simulink model "gm_smartCart3"  (R2016a)
settings: Solver=FixedStepDiscrete  StartTime=0.0  StopTime=600000  FixedStep=1  RelTol=1e-3
libraries: simulink x56, hdlsllib x28
(part 1 of 2)
settings Model: Creator=Admin  LastModifiedBy=Admin
settings OptimizationCC: BlockReduction=off  ConditionallyExecuteInputs=off  DefaultParameterBehavior=Inlined
settings DebuggingCC: AlgebraicLoopMsg=error  InheritedTsInSrcMsg=none
settings HardwareCC: ProdBitPerPointer=32  ProdLargestAtomicFloat=None  ProdIntDivRoundTo=Undefined  ProdEndianess=Unspecified  ProdWordSize=32  ProdHWDeviceType=ASIC/FPGA->ASIC/FPGA  ProdEqTarget=off

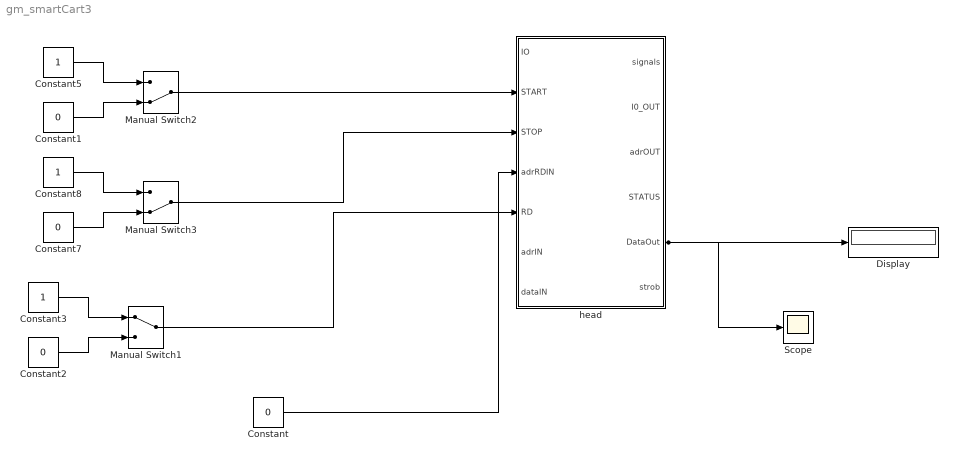
== system gm_smartCart3 ==
  Constant : Constant  Value=0  OutDataTypeStr=uint8
  Constant1 : Constant  Value=0  OutDataTypeStr=boolean
  Constant2 : Constant  Value=0  OutDataTypeStr=boolean
  Constant3 : Constant  OutDataTypeStr=boolean
  Constant5 : Constant  OutDataTypeStr=boolean
  Constant7 : Constant  Value=0  OutDataTypeStr=boolean
  Constant8 : Constant  OutDataTypeStr=boolean
  Display : Display
  Manual Switch1 : ManualSwitch
  Manual Switch2 : ManualSwitch  CurrentSetting=0
  Manual Switch3 : ManualSwitch  CurrentSetting=0
  Scope : Scope
  head : Subsystem  TreatAsAtomicUnit=on
  wires:
  Manual Switch1/1 -> head/5(RD)
  head/5(DataOut) -> Display/1, Scope/1
  Constant2/1 -> Manual Switch1/2
  Constant3/1 -> Manual Switch1/1
  Constant/1 -> head/4(adrRDIN)
  Manual Switch3/1 -> head/3(STOP)
  Constant7/1 -> Manual Switch3/2
  Constant8/1 -> Manual Switch3/1
  Manual Switch2/1 -> head/2(START)
  Constant1/1 -> Manual Switch2/2
  Constant5/1 -> Manual Switch2/1

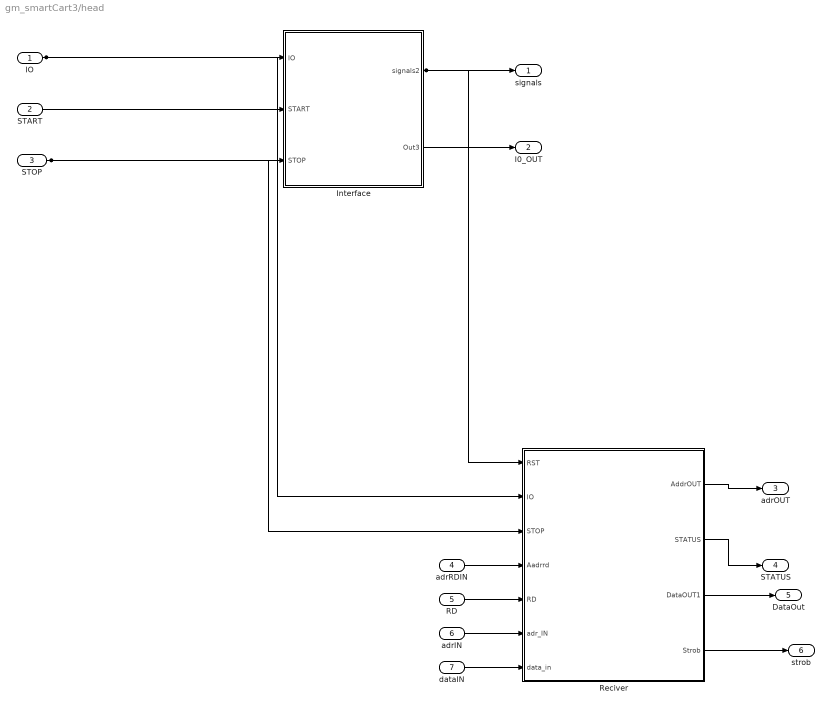
== system gm_smartCart3/head ==
  IO : Inport  OutDataTypeStr=boolean
  START : Inport  Port=2  OutDataTypeStr=boolean  SampleTime=1
  STOP : Inport  Port=3  OutDataTypeStr=boolean  SampleTime=1
  adrRDIN : Inport  Port=4  OutDataTypeStr=uint8
  RD : Inport  Port=5  OutDataTypeStr=boolean  SampleTime=1
  adrIN : Inport  Port=6  OutDataTypeStr=uint8
  dataIN : Inport  Port=7  OutDataTypeStr=uint32
  Interface : Subsystem
  Reciver : Subsystem
  signals : Outport  OutDataTypeStr=fixdt(1,4,0)
  I0_OUT : Outport  Port=2  OutDataTypeStr=boolean
  adrOUT : Outport  Port=3  OutDataTypeStr=uint8
  STATUS : Outport  Port=4  OutDataTypeStr=uint32
  DataOut : Outport  Port=5  OutDataTypeStr=uint8
  strob : Outport  Port=6  OutDataTypeStr=boolean
  wires:
  IO/1 -> Reciver/2(IO), Interface/1(IO)
  START/1 -> Interface/2(START)
  STOP/1 -> Reciver/3(STOP), Interface/3(STOP)
  adrRDIN/1 -> Reciver/4(Aadrrd)
  RD/1 -> Reciver/5(RD)
  adrIN/1 -> Reciver/6(adr_IN)
  dataIN/1 -> Reciver/7(data_in)
  Interface/1(signals2) -> Reciver/1(RST), signals/1
  Interface/2(Out3) -> I0_OUT/1
  Reciver/1(AddrOUT) -> adrOUT/1
  Reciver/2(STATUS) -> STATUS/1
  Reciver/3(DataOUT1) -> DataOut/1
  Reciver/4(Strob) -> strob/1

== system gm_smartCart3/head/Interface ==
  IO : Inport  OutDataTypeStr=boolean
  START : Inport  Port=2  OutDataTypeStr=boolean  SampleTime=1
  STOP : Inport  Port=3  OutDataTypeStr=boolean  SampleTime=1
  ColdStart : Subsystem
  ColdStop2 : Subsystem
  Head2 : Subsystem
  MUX2 : Subsystem
  Swith_signal2 : Subsystem
  signals2 : Outport  OutDataTypeStr=fixdt(1,4,0)  InitialOutput=0
  Out3 : Outport  Port=2  OutDataTypeStr=boolean  InitialOutput=0
  wires:
  IO/1 -> Out3/1, ColdStart/1(Reqest)
  START/1 -> Head2/3(START)
  STOP/1 -> Head2/4(STOP)
  ColdStart/1(DataOUT) -> MUX2/5(DAT_ST1)
  ColdStart/2(Signal) -> MUX2/2(DATA_0)
  ColdStart/3(ADR_OUT) -> MUX2/4(ADR_ST)
  ColdStop2/1(DataOUT) -> MUX2/7(DAT_STOP)
  ColdStop2/2(Signal) -> MUX2/3(DATA_1)
  ColdStop2/3(ADR_OUT) -> MUX2/6(ADR_STOP)
  Head2/1(AdrOut) -> Swith_signal2/1(Adr), ColdStart/2(Addr), ColdStop2/1(Addr)
  Head2/2(DataOut) -> Swith_signal2/2(Data), ColdStart/3(Data), ColdStop2/2(Data)
  MUX2/1(Signals) -> signals2/1
  MUX2/2(ADR_OUT) -> Head2/1(ADR_IN)
  MUX2/3(DATA_OUT1) -> Head2/2(DataIN)
  Swith_signal2/1(OutAddr) -> MUX2/1(ADR)

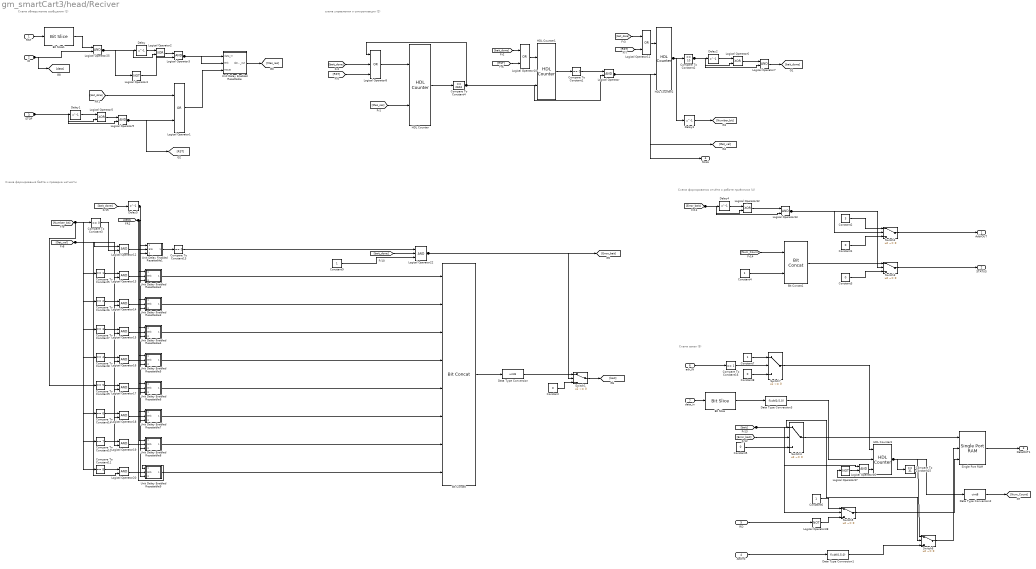
== system gm_smartCart3/head/Reciver ==
  note: Схема обнаружение сообщения (1)
  note: cхема управления и синхронизации (2)
  note: Схема формирования отчёта о работе приёмника (4)
  note: Схема связи (5)
  note: Cхема формирования байта и проверка четности
  RST : Inport  OutDataTypeStr=fixdt(1,4,0)  SampleTime=1
  IO : Inport  Port=2  OutDataTypeStr=boolean
  STOP : Inport  Port=3  OutDataTypeStr=boolean  SampleTime=1
  Aadrrd : Inport  Port=4  OutDataTypeStr=uint8
  RD : Inport  Port=5  OutDataTypeStr=boolean  SampleTime=1
  adr_IN : Inport  Port=6  OutDataTypeStr=uint8
  data_in : Inport  Port=7  OutDataTypeStr=uint32
  Bit Concat : hdlsllib/HDL Operations/Bit Concat  numInputs=8
  Bit Concat1 : hdlsllib/HDL Operations/Bit Concat  numInputs=2
  Bit Slice : hdlsllib/HDL Operations/Bit Slice  lidx=5  ridx=0
  Bit Slice1 : hdlsllib/HDL Operations/Bit Slice  lidx=3  ridx=3
  Compare To Constant1 : simulink/Logic and Bit Operations/Compare To Constant  relop===  const=0  OutDataTypeStr=boolean
  Compare To Constant10 : simulink/Logic and Bit Operations/Compare To Constant  relop===  const=7  OutDataTypeStr=boolean
  Compare To Constant11 : simulink/Logic and Bit Operations/Compare To Constant  relop===  const=8  OutDataTypeStr=boolean
  Compare To Constant13 : simulink/Logic and Bit Operations/Compare To Constant  relop===  const=0  OutDataTypeStr=boolean
  Compare To Constant14 : simulink/Logic and Bit Operations/Compare To Constant  relop===  const=6  OutDataTypeStr=boolean
  Compare To Constant15 : simulink/Logic and Bit Operations/Compare To Constant  relop===  const=31  OutDataTypeStr=boolean
  Compare To Constant16 : simulink/Logic and Bit Operations/Compare To Constant  relop===  const=1  OutDataTypeStr=boolean
  Compare To Constant2 : simulink/Logic and Bit Operations/Compare To Constant  relop===  const=10  OutDataTypeStr=boolean
  Compare To Constant3 : simulink/Logic and Bit Operations/Compare To Constant  relop===  const=0  OutDataTypeStr=boolean
  Compare To Constant4 : simulink/Logic and Bit Operations/Compare To Constant  relop===  const=2604  OutDataTypeStr=boolean
  Compare To Constant5 : simulink/Logic and Bit Operations/Compare To Constant  relop===  const=1  OutDataTypeStr=boolean
  Compare To Constant6 : simulink/Logic and Bit Operations/Compare To Constant  relop===  const=2  OutDataTypeStr=boolean
  Compare To Constant7 : simulink/Logic and Bit Operations/Compare To Constant  relop===  const=3  OutDataTypeStr=boolean
  Compare To Constant8 : simulink/Logic and Bit Operations/Compare To Constant  relop===  const=4  OutDataTypeStr=boolean
  Compare To Constant9 : simulink/Logic and Bit Operations/Compare To Constant  relop===  const=5  OutDataTypeStr=boolean
  Constant : Constant  Value=0  OutDataTypeStr=uint8
  Constant1 : Constant  Value=0  OutDataTypeStr=uint8
  Constant2 : Constant  Value=3  OutDataTypeStr=uint8
  Constant3 : Constant  Value=0  OutDataTypeStr=uint32
  Constant4 : Constant  OutDataTypeStr=boolean
  Constant5 : Constant  Value=0  OutDataTypeStr=uint8  SampleTime=-1
  Constant6 : Constant  OutDataTypeStr=boolean  SampleTime=-1
  Constant7 : Constant  OutDataTypeStr=boolean
  Constant8 : Constant  Value=0  OutDataTypeStr=boolean
  Constant9 : Constant  OutDataTypeStr=boolean
  Data Type Conversion : DataTypeConversion  OutDataTypeStr=uint8
  Data Type Conversion1 : DataTypeConversion  OutDataTypeStr=fixdt(0,5,0)
  Data Type Conversion2 : DataTypeConversion  OutDataTypeStr=uint8
  Data Type Conversion3 : DataTypeConversion  OutDataTypeStr=fixdt(0,5,0)
  Delay{,1..5} (6 alike) : Delay  DelayLength=1  InitialCondition=0
  HDL Counter : hdlsllib/HDL Operations/HDL Counter  CountType=Free running  CountInit=0  CountStep=1  CountMax=1  CountFromType=Initial value  CountFrom=0  CountResetPort=on  CountLoadPort=off  CountEnbPort=on  CountDirPort=off  CountDataType=Unsigned  CountWordLen=13  CountFracLen=0  CountSampTime=1
  HDL Counter1 : hdlsllib/HDL Operations/HDL Counter  CountType=Free running  CountInit=0  CountStep=1  CountMax=1  CountFromType=Initial value  CountFrom=0  CountResetPort=on  CountLoadPort=off  CountEnbPort=on  CountDirPort=off  CountDataType=Unsigned  CountWordLen=1  CountFracLen=0  CountSampTime=1
  HDL Counter2 : hdlsllib/HDL Operations/HDL Counter  CountType=Count limited  CountInit=0  CountStep=1  CountMax=10  CountFromType=Initial value  CountFrom=0  CountResetPort=on  CountLoadPort=off  CountEnbPort=on  CountDirPort=off  CountDataType=Unsigned  CountWordLen=4  CountFracLen=0  CountSampTime=1
  HDL Counter3 : hdlsllib/HDL Operations/HDL Counter  CountType=Free running  CountInit=0  CountStep=1  CountMax=1  CountFromType=Initial value  CountFrom=0  CountResetPort=off  CountLoadPort=on  CountEnbPort=on  CountDirPort=off  CountDataType=Unsigned  CountWordLen=5  CountFracLen=0  CountSampTime=1
  Logical Operator{,3,7,9,12..20,25,33,36} (16 alike) : Logic  AllPortsSameDT=off  OutDataTypeStr=boolean
  Logical Operator1 : Logic  Operator=OR  AllPortsSameDT=off  OutDataTypeStr=boolean
  Logical Operator10 : Logic  Operator=OR  AllPortsSameDT=off  OutDataTypeStr=boolean
  Logical Operator11 : Logic  Operator=OR  AllPortsSameDT=off  OutDataTypeStr=boolean
  Logical Operator{2,5..6,32} (4 alike) : Logic  Operator=XOR  AllPortsSameDT=off  OutDataTypeStr=boolean
  Logical Operator22 : Logic  Inputs=3  AllPortsSameDT=off  OutDataTypeStr=boolean
  Logical Operator37 : Logic  Operator=NOT  AllPortsSameDT=off  OutDataTypeStr=boolean
  Logical Operator38 : Logic  Operator=NOT  AllPortsSameDT=off  OutDataTypeStr=boolean
  Logical Operator4 : Logic  Operator=NOT  AllPortsSameDT=off  OutDataTypeStr=boolean
  Logical Operator8 : Logic  Operator=OR  Inputs=3  AllPortsSameDT=off  OutDataTypeStr=boolean
  Single Port RAM : hdlsllib/HDL Operations/Single Port RAM  ram_size=5  dout_type=Old data
  Switch{1..7} (7 alike) : Switch  Criteria=u2 ~= 0
  Unit Delay Enabled Resettable : Subsystem
  Unit Delay Enabled Resettable1 : Subsystem
  Unit Delay Enabled Resettable2 : Subsystem
  Unit Delay Enabled Resettable3 : Subsystem
  Unit Delay Enabled Resettable4 : Subsystem
  Unit Delay Enabled Resettable5 : Subsystem
  Unit Delay Enabled Resettable6 : Subsystem
  Unit Delay Enabled Resettable7 : Subsystem
  Unit Delay Enabled Resettable8 : Subsystem
  Unit Delay Enabled Resettable9 : Subsystem
  AddrOUT : Outport  OutDataTypeStr=uint8
  STATUS : Outport  Port=2  OutDataTypeStr=uint32
  DataOUT1 : Outport  Port=3  OutDataTypeStr=uint8
  Strob : Outport  Port=4  OutDataTypeStr=boolean
  wires:
  RST/1 -> Bit Slice1/1
  IO/1 -> Logical Operator25/2, [data]
  STOP/1 -> Logical Operator9/2, Logical Operator5/2, Delay1/1
  Aadrrd/1 -> Data Type Conversion1/1
  RD/1 -> Logical Operator38/1
  adr_IN/1 -> Compare To Constant16/1
  data_in/1 -> Bit Slice/1
  Bit Concat/1 -> Data Type Conversion/1
  Bit Concat1/1 -> Switch3/1
  Bit Slice/1 -> Data Type Conversion3/1
  Bit Slice1/1 -> Logical Operator25/1
  Compare To Constant1/1 -> Logical Operator/1
  Compare To Constant10/1 -> Logical Operator19/1
  Compare To Constant11/1 -> Logical Operator20/1
  Compare To Constant13/1 -> Logical Operator22/1
  Compare To Constant14/1 -> Logical Operator18/1
  Compare To Constant15/1 -> Logical Operator37/1
  Compare To Constant16/1 -> Switch7/2
  Compare To Constant2/1 -> Logical Operator7/2, Logical Operator6/2, Delay2/1
  Compare To Constant3/1 -> Logical Operator12/2
  Compare To Constant4/1 -> Logical Operator8/1, Logical Operator/2, HDL Counter1/2
  Compare To Constant5/1 -> Logical Operator13/1
  Compare To Constant6/1 -> Logical Operator14/1
  Compare To Constant7/1 -> Logical Operator15/1
  Compare To Constant8/1 -> Logical Operator16/1
  Compare To Constant9/1 -> Logical Operator17/1
  Constant/1 -> Switch1/3
  Constant1/1 -> Switch2/3
  Constant2/1 -> Switch2/1
  Constant3/1 -> Switch3/3
  Constant4/1 -> Bit Concat1/2
  Constant5/1 -> Switch4/3
  Constant6/1 -> Switch5/1
  Constant7/1 -> Switch7/1
  Constant8/1 -> Switch7/3
  Constant9/1 -> Logical Operator22/3
  Data Type Conversion/1 -> Switch1/1
  Data Type Conversion1/1 -> Switch6/3
  Data Type Conversion2/1 -> [Num_Count]
  Data Type Conversion3/1 -> HDL Counter3/2
  Delay/1 -> Logical Operator2/1
  Delay1/1 -> Logical Operator5/1
  Delay2/1 -> Logical Operator6/1
  Delay3/1 -> [Number_bit]
  Delay4/1 -> Logical Operator32/1
  Delay5/1 -> Unit Delay Enabled Resettable9/3(Reset), Unit Delay Enabled Resettable8/3(Reset), Unit Delay Enabled Resettable7/3(Reset), Unit Delay Enabled Resettable6/3(Reset), Unit Delay Enabled Resettable5/3(Reset), Unit Delay Enabled Resettable4/3(Reset), Unit Delay Enabled Resettable3/3(Reset), Unit Delay Enabled Resettable2/3(Reset), Unit Delay Enabled Resettable1/3(Reset)
  [bait_done] -> Logical Operator1/1
  [data] -> Unit Delay Enabled Resettable9/1(data_in), Unit Delay Enabled Resettable8/1(data_in), Unit Delay Enabled Resettable7/1(data_in), Unit Delay Enabled Resettable6/1(data_in), Unit Delay Enabled Resettable5/1(data_in), Unit Delay Enabled Resettable4/1(data_in), Unit Delay Enabled Resettable3/1(data_in), Unit Delay Enabled Resettable2/1(data_in), Unit Delay Enabled Resettable1/1(data_in)
  [Mes_res] -> HDL Counter/2
  [bait_done] -> Logical Operator22/2
  [Error_bait] -> Logical Operator33/2, Logical Operator32/2, Delay4/1
  [Error_bait] -> Switch4/2
  [bait] -> Switch6/2, Switch5/2, Switch4/1, Logical Operator36/1
  [Num_Count] -> Bit Concat1/1
  [bait_done] -> Delay5/1
  [bait_done] -> Logical Operator10/1
  [bait_done] -> Logical Operator11/1
  [bait_done] -> Logical Operator8/2
  [RST] -> Logical Operator8/3
  [RST] -> Logical Operator10/2
  [RST] -> Logical Operator11/2
  [Get_val] -> Logical Operator20/2, Logical Operator19/2, Logical Operator18/2, Logical Operator17/2, Logical Operator16/2, Logical Operator15/2, Logical Operator14/2, Logical Operator13/2, Logical Operator12/1
  [Number_bit] -> Compare To Constant9/1, Compare To Constant8/1, Compare To Constant7/1, Compare To Constant6/1, Compare To Constant5/1, Compare To Constant3/1, Compare To Constant14/1, Compare To Constant11/1, Compare To Constant10/1
  HDL Counter/1 -> Compare To Constant4/1
  HDL Counter1/1 -> Compare To Constant1/1
  HDL Counter2/1 -> Compare To Constant2/1, Delay3/1
  HDL Counter3/1 -> Switch6/1, Data Type Conversion2/1, Compare To Constant15/1
  Logical Operator/1 -> HDL Counter2/2, [Get_val], Strob/1
  Logical Operator1/1 -> Unit Delay Enabled Resettable/3(Reset)
  Logical Operator10/1 -> HDL Counter1/1
  Logical Operator11/1 -> HDL Counter2/1
  Logical Operator12/1 -> Unit Delay Enabled Resettable1/2(Enb)
  Logical Operator13/1 -> Unit Delay Enabled Resettable2/2(Enb)
  Logical Operator14/1 -> Unit Delay Enabled Resettable3/2(Enb)
  Logical Operator15/1 -> Unit Delay Enabled Resettable4/2(Enb)
  Logical Operator16/1 -> Unit Delay Enabled Resettable5/2(Enb)
  Logical Operator17/1 -> Unit Delay Enabled Resettable6/2(Enb)
  Logical Operator18/1 -> Unit Delay Enabled Resettable7/2(Enb)
  Logical Operator19/1 -> Unit Delay Enabled Resettable8/2(Enb)
  Logical Operator2/1 -> Logical Operator3/1
  Logical Operator20/1 -> Unit Delay Enabled Resettable9/2(Enb)
  Logical Operator22/1 -> Switch1/2, [Error_bait]
  Logical Operator25/1 -> Logical Operator4/1, Logical Operator2/2, Delay/1
  Logical Operator3/1 -> Unit Delay Enabled Resettable/2(Enb), Unit Delay Enabled Resettable/1(data_in)
  Logical Operator32/1 -> Logical Operator33/1
  Logical Operator33/1 -> Switch3/2, Switch2/2
  Logical Operator36/1 -> HDL Counter3/3
  Logical Operator37/1 -> Logical Operator36/2
  Logical Operator38/1 -> Switch5/3
  Logical Operator4/1 -> Logical Operator3/2
  Logical Operator5/1 -> Logical Operator9/1
  Logical Operator6/1 -> Logical Operator7/1
  Logical Operator7/1 -> [bait_done]
  Logical Operator8/1 -> HDL Counter/1
  Logical Operator9/1 -> Logical Operator1/2, [RST]
  Single Port RAM/1 -> DataOUT1/1
  Switch1/1 -> [bait]
  Switch2/1 -> AddrOUT/1
  Switch3/1 -> STATUS/1
  Switch4/1 -> Single Port RAM/1
  Switch5/1 -> Single Port RAM/3
  Switch6/1 -> Single Port RAM/2
  Switch7/1 -> HDL Counter3/1
  Unit Delay Enabled Resettable/1(data_out) -> [Mes_res]
  Unit Delay Enabled Resettable1/1(data_out) -> Compare To Constant13/1
  Unit Delay Enabled Resettable2/1(data_out) -> Bit Concat/1
  Unit Delay Enabled Resettable3/1(data_out) -> Bit Concat/2
  Unit Delay Enabled Resettable4/1(data_out) -> Bit Concat/3
  Unit Delay Enabled Resettable5/1(data_out) -> Bit Concat/4
  Unit Delay Enabled Resettable6/1(data_out) -> Bit Concat/5
  Unit Delay Enabled Resettable7/1(data_out) -> Bit Concat/6
  Unit Delay Enabled Resettable8/1(data_out) -> Bit Concat/7
  Unit Delay Enabled Resettable9/1(data_out) -> Bit Concat/8

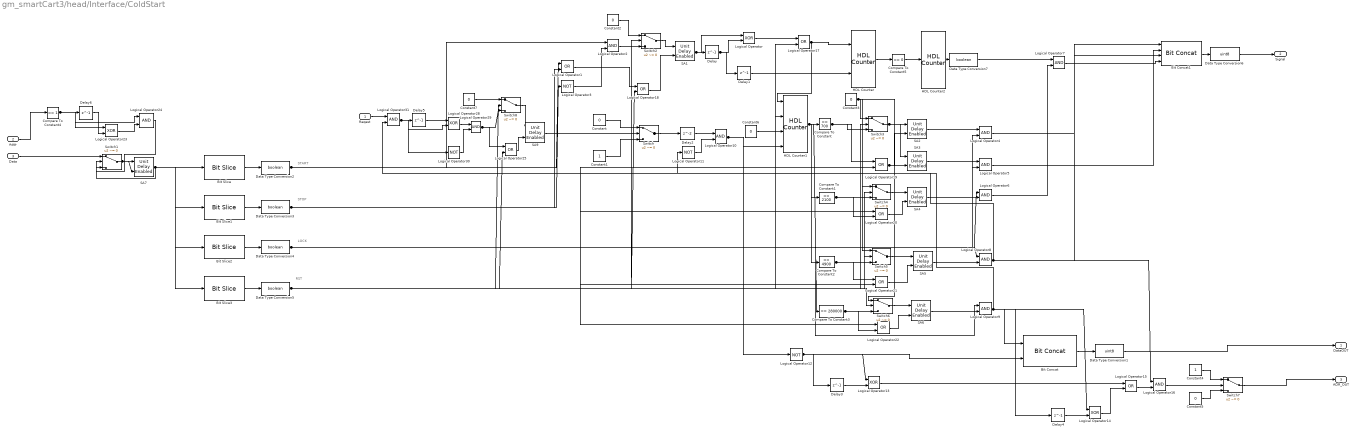
== system gm_smartCart3/head/Interface/ColdStart ==
  note: LOCK
  note: STOP
  note: START
  note: RST
  Reqest : Inport  OutDataTypeStr=boolean
  Addr : Inport  Port=2  OutDataTypeStr=uint8  SampleTime=1
  Data : Inport  Port=3  OutDataTypeStr=uint8  SampleTime=1
  Bit Concat : hdlsllib/HDL Operations/Bit Concat  numInputs=2
  Bit Concat1 : hdlsllib/HDL Operations/Bit Concat  numInputs=4
  Bit Slice : hdlsllib/HDL Operations/Bit Slice  lidx=3  ridx=3
  Bit Slice1 : hdlsllib/HDL Operations/Bit Slice  lidx=2  ridx=2
  Bit Slice2 : hdlsllib/HDL Operations/Bit Slice  lidx=1  ridx=1
  Bit Slice3 : hdlsllib/HDL Operations/Bit Slice  lidx=0  ridx=0
  Compare To Constant : simulink/Logic and Bit Operations/Compare To Constant  relop===  const=700  OutDataTypeStr=boolean
  Compare To Constant1 : simulink/Logic and Bit Operations/Compare To Constant  relop===  const=2100  OutDataTypeStr=boolean
  Compare To Constant2 : simulink/Logic and Bit Operations/Compare To Constant  relop===  const=4900  OutDataTypeStr=boolean
  Compare To Constant3 : simulink/Logic and Bit Operations/Compare To Constant  relop===  const=280000  OutDataTypeStr=boolean
  Compare To Constant4 : simulink/Logic and Bit Operations/Compare To Constant  relop===  const=1  OutDataTypeStr=boolean
  Compare To Constant5 : simulink/Logic and Bit Operations/Compare To Constant  relop===  const=0  OutDataTypeStr=boolean
  Constant{,2..3,7} (4 alike) : Constant  Value=0  OutDataTypeStr=boolean
  Constant1 : Constant  OutDataTypeStr=boolean
  Constant4 : Constant  OutDataTypeStr=uint8
  Constant5 : Constant  Value=0  OutDataTypeStr=uint8
  Constant6 : Constant  Value=0  OutDataTypeStr=fixdt(0,32,0)
  Data Type Conversion1 : DataTypeConversion  OutDataTypeStr=uint8
  Data Type Conversion{2..5,7} (5 alike) : DataTypeConversion  OutDataTypeStr=boolean
  Data Type Conversion6 : DataTypeConversion  OutDataTypeStr=uint8
  Delay{,1,3..6} (6 alike) : Delay  DelayLength=1  InitialCondition=0
  Delay2 : Delay  InitialCondition=0
  HDL Counter : hdlsllib/HDL Operations/HDL Counter  CountType=Count limited  CountInit=0  CountStep=1  CountMax=6  CountFromType=Initial value  CountFrom=0  CountResetPort=on  CountLoadPort=off  CountEnbPort=on  CountDirPort=off  CountDataType=Unsigned  CountWordLen=3  CountFracLen=0  CountSampTime=277e-9
  HDL Counter1 : hdlsllib/HDL Operations/HDL Counter  CountType=Count limited  CountInit=0  CountStep=1  CountMax=40000  CountFromType=Initial value  CountFrom=0  CountResetPort=on  CountLoadPort=on  CountEnbPort=on  CountDirPort=off  CountDataType=Unsigned  CountWordLen=32  CountFracLen=0  CountSampTime=277e-9
  HDL Counter2 : hdlsllib/HDL Operations/HDL Counter  CountType=Free running  CountInit=0  CountStep=1  CountMax=5  CountFromType=Initial value  CountFrom=0  CountResetPort=off  CountLoadPort=off  CountEnbPort=on  CountDirPort=off  CountDataType=Unsigned  CountWordLen=1  CountFracLen=0  CountSampTime=277e-9
  Logical Operator{,13..14,23,28} (5 alike) : Logic  Operator=XOR  AllPortsSameDT=off  OutDataTypeStr=boolean
  Logical Operator{1,15,17..22,25} (9 alike) : Logic  Operator=OR  AllPortsSameDT=off  OutDataTypeStr=boolean
  Logical Operator{2,4..10,16,24,29,31} (12 alike) : Logic  AllPortsSameDT=off  OutDataTypeStr=boolean
  Logical Operator{3,11..12,30} (4 alike) : Logic  Operator=NOT  AllPortsSameDT=off  OutDataTypeStr=boolean
  SA{1..7,9} (8 alike) : simulink/Additional Math & Discrete/Additional Discrete/Unit Delay Enabled  vinit=0  tsamp=-1
  Switch{,1..8} (9 alike) : Switch  Criteria=u2 ~= 0
  DataOUT : Outport  OutDataTypeStr=uint8
  Signal : Outport  Port=2  OutDataTypeStr=uint8
  ADR_OUT : Outport  Port=3  OutDataTypeStr=uint8
  wires:
  Reqest/1 -> Logical Operator31/1
  Addr/1 -> Compare To Constant4/1
  Data/1 -> Switch1/1
  Bit Concat/1 -> Data Type Conversion1/1
  Bit Concat1/1 -> Data Type Conversion6/1
  Bit Slice/1 -> Data Type Conversion2/1
  Bit Slice1/1 -> Data Type Conversion3/1
  Bit Slice2/1 -> Data Type Conversion4/1
  Bit Slice3/1 -> Data Type Conversion5/1
  Compare To Constant/1 -> Switch3/3, Logical Operator19/1
  Compare To Constant1/1 -> Switch4/3, Logical Operator20/2
  Compare To Constant2/1 -> Switch5/3, Logical Operator21/1
  Compare To Constant3/1 -> Switch6/3, Logical Operator22/2
  Compare To Constant4/1 -> Logical Operator24/1, Logical Operator23/1, Delay6/1
  Compare To Constant5/1 -> HDL Counter2/1
  Constant/1 -> Switch/1
  Constant1/1 -> Switch/3
  Constant2/1 -> Switch2/1
  Constant3/1 -> Switch6/1, Switch5/1, Switch4/1, Switch3/1
  Constant4/1 -> Switch7/1
  Constant5/1 -> Switch7/3
  Constant6/1 -> HDL Counter1/3
  Constant7/1 -> Switch8/1
  Data Type Conversion1/1 -> DataOUT/1
  Data Type Conversion2/1 -> Logical Operator2/1, Logical Operator1/1
  Data Type Conversion3/1 -> Logical Operator3/1, Logical Operator1/2
  Data Type Conversion4/1 -> Logical Operator9/1, Logical Operator8/1, Logical Operator6/1, Logical Operator5/2, Logical Operator4/2
  Data Type Conversion5/1 -> Switch8/2, Switch6/2, Switch5/2, Switch4/2, Switch3/2, Switch2/2, Logical Operator25/2, Logical Operator22/1, Logical Operator21/2, Logical Operator20/1, Logical Operator19/2, Logical Operator18/2, Logical Operator17/2, HDL Counter1/2
  Data Type Conversion6/1 -> Signal/1
  Data Type Conversion7/1 -> Logical Operator7/1
  Delay/1 -> Logical Operator/2, Delay1/1
  Delay1/1 -> HDL Counter/2
  Delay2/1 -> Logical Operator10/1
  Delay3/1 -> Logical Operator13/2
  Delay4/1 -> Logical Operator14/2
  Delay5/1 -> Logical Operator28/1
  Delay6/1 -> Logical Operator23/2
  HDL Counter/1 -> Compare To Constant5/1
  HDL Counter1/1 -> Compare To Constant3/1, Compare To Constant2/1, Compare To Constant1/1, Compare To Constant/1
  HDL Counter2/1 -> Data Type Conversion7/1
  Logical Operator/1 -> Logical Operator17/1
  Logical Operator1/1 -> Logical Operator18/1
  Logical Operator10/1 -> Logical Operator12/1, HDL Counter1/4
  Logical Operator11/1 -> Logical Operator10/2
  Logical Operator12/1 -> Logical Operator13/1, Bit Concat/2, Delay3/1
  Logical Operator13/1 -> Logical Operator15/1
  Logical Operator14/1 -> Logical Operator15/2
  Logical Operator15/1 -> Logical Operator16/2
  Logical Operator16/1 -> Switch7/2
  Logical Operator17/1 -> HDL Counter1/1, HDL Counter/1
  Logical Operator18/1 -> SA1/2
  Logical Operator19/1 -> SA3/2, SA2/2
  Logical Operator2/1 -> Switch2/3
  Logical Operator20/1 -> SA4/2
  Logical Operator21/1 -> SA5/2
  Logical Operator22/1 -> SA6/2
  Logical Operator23/1 -> Logical Operator24/2
  Logical Operator24/1 -> Switch1/2
  Logical Operator25/1 -> SA9/2
  Logical Operator28/1 -> Logical Operator29/1
  Logical Operator29/1 -> Switch8/3, Logical Operator25/1
  Logical Operator3/1 -> Logical Operator2/2
  Logical Operator30/1 -> Logical Operator29/2
  Logical Operator31/1 -> Logical Operator30/1, Logical Operator28/2, Delay5/1
  Logical Operator4/1 -> Bit Concat1/3
  Logical Operator5/1 -> Bit Concat1/2
  Logical Operator6/1 -> Logical Operator7/2
  Logical Operator7/1 -> Bit Concat1/4
  Logical Operator8/1 -> Logical Operator31/2, Logical Operator16/1, Bit Concat1/1
  Logical Operator9/1 -> Logical Operator14/1, Logical Operator11/1, Bit Concat/1, Delay4/1
  SA1/1 -> Logical Operator/1, Delay/1
  SA2/1 -> Logical Operator4/1
  SA3/1 -> Logical Operator5/1
  SA4/1 -> Logical Operator6/2
  SA5/1 -> Logical Operator8/2
  SA6/1 -> Logical Operator9/2
  SA7/1 -> Switch1/3, Bit Slice3/1, Bit Slice2/1, Bit Slice1/1, Bit Slice/1
  SA9/1 -> Switch/2
  Switch/1 -> Delay2/1
  Switch1/1 -> SA7/2, SA7/1
  Switch2/1 -> SA1/1
  Switch3/1 -> SA3/1, SA2/1
  Switch4/1 -> SA4/1
  Switch5/1 -> SA5/1
  Switch6/1 -> SA6/1
  Switch7/1 -> ADR_OUT/1
  Switch8/1 -> SA9/1

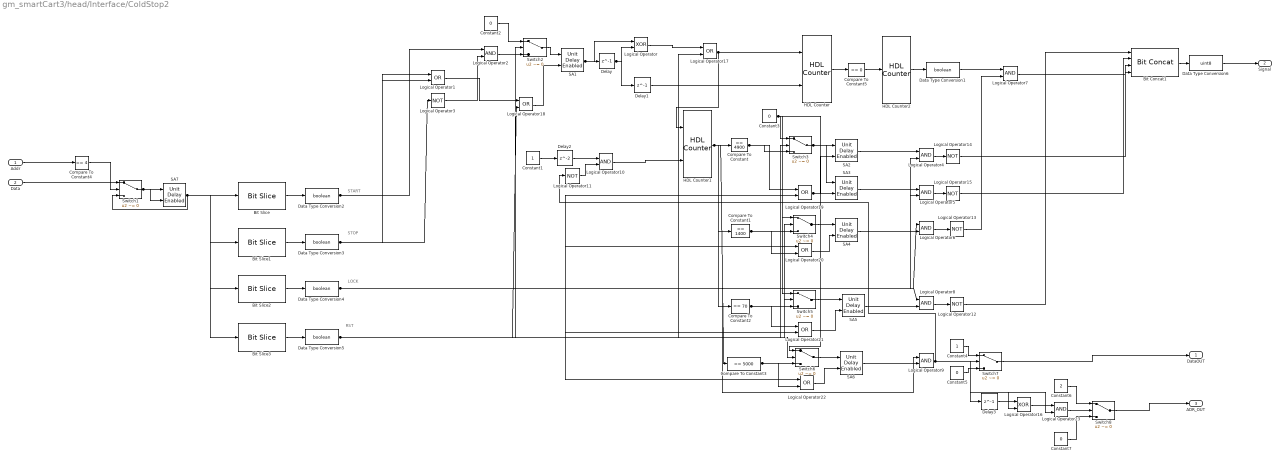
== system gm_smartCart3/head/Interface/ColdStop2 ==
  note: LOCK
  note: STOP
  note: START
  note: RST
  Addr : Inport  OutDataTypeStr=uint8  SampleTime=1
  Data : Inport  Port=2  OutDataTypeStr=uint8  SampleTime=1
  Bit Concat1 : hdlsllib/HDL Operations/Bit Concat  numInputs=4
  Bit Slice : hdlsllib/HDL Operations/Bit Slice  lidx=3  ridx=3
  Bit Slice1 : hdlsllib/HDL Operations/Bit Slice  lidx=2  ridx=2
  Bit Slice2 : hdlsllib/HDL Operations/Bit Slice  lidx=1  ridx=1
  Bit Slice3 : hdlsllib/HDL Operations/Bit Slice  lidx=0  ridx=0
  Compare To Constant : simulink/Logic and Bit Operations/Compare To Constant  relop===  const=4900  OutDataTypeStr=boolean
  Compare To Constant1 : simulink/Logic and Bit Operations/Compare To Constant  relop===  const=1400  OutDataTypeStr=boolean
  Compare To Constant2 : simulink/Logic and Bit Operations/Compare To Constant  relop===  const=70  OutDataTypeStr=boolean
  Compare To Constant3 : simulink/Logic and Bit Operations/Compare To Constant  relop===  const=5000  OutDataTypeStr=boolean
  Compare To Constant4 : simulink/Logic and Bit Operations/Compare To Constant  relop===  const=4  OutDataTypeStr=boolean
  Compare To Constant5 : simulink/Logic and Bit Operations/Compare To Constant  relop===  const=0  OutDataTypeStr=boolean
  Constant1 : Constant  OutDataTypeStr=boolean
  Constant2 : Constant  Value=0  OutDataTypeStr=boolean
  Constant3 : Constant  Value=0  OutDataTypeStr=boolean
  Constant4 : Constant  OutDataTypeStr=uint8
  Constant5 : Constant  Value=0  OutDataTypeStr=uint8
  Constant6 : Constant  Value=2  OutDataTypeStr=uint8
  Constant7 : Constant  Value=0  OutDataTypeStr=uint8
  Data Type Conversion{1..5} (5 alike) : DataTypeConversion  OutDataTypeStr=boolean
  Data Type Conversion6 : DataTypeConversion  OutDataTypeStr=uint8
  Delay : Delay  DelayLength=1  InitialCondition=0
  Delay1 : Delay  DelayLength=1  InitialCondition=0
  Delay2 : Delay  InitialCondition=0
  Delay3 : Delay  DelayLength=1  InitialCondition=0
  HDL Counter : hdlsllib/HDL Operations/HDL Counter  CountType=Count limited  CountInit=0  CountStep=1  CountMax=6  CountFromType=Initial value  CountFrom=0  CountResetPort=on  CountLoadPort=off  CountEnbPort=on  CountDirPort=off  CountDataType=Unsigned  CountWordLen=3  CountFracLen=0  CountSampTime=277e-9
  HDL Counter1 : hdlsllib/HDL Operations/HDL Counter  CountType=Count limited  CountInit=0  CountStep=1  CountMax=40000  CountFromType=Initial value  CountFrom=0  CountResetPort=on  CountLoadPort=off  CountEnbPort=on  CountDirPort=off  CountDataType=Unsigned  CountWordLen=32  CountFracLen=0  CountSampTime=277e-9
  HDL Counter2 : hdlsllib/HDL Operations/HDL Counter  CountType=Free running  CountInit=0  CountStep=1  CountMax=6  CountFromType=Initial value  CountFrom=0  CountResetPort=off  CountLoadPort=off  CountEnbPort=on  CountDirPort=off  CountDataType=Unsigned  CountWordLen=1  CountFracLen=0  CountSampTime=277e-9
  Logical Operator : Logic  Operator=XOR  AllPortsSameDT=off  OutDataTypeStr=boolean
  Logical Operator{1,17..22} (7 alike) : Logic  Operator=OR  AllPortsSameDT=off  OutDataTypeStr=boolean
  Logical Operator{2,4..10,23} (9 alike) : Logic  AllPortsSameDT=off  OutDataTypeStr=boolean
  Logical Operator{3,11..15} (6 alike) : Logic  Operator=NOT  AllPortsSameDT=off  OutDataTypeStr=boolean
  Logical Operator16 : Logic  Operator=XOR  AllPortsSameDT=off  OutDataTypeStr=boolean
  SA{1..7} (7 alike) : simulink/Additional Math & Discrete/Additional Discrete/Unit Delay Enabled  vinit=0  tsamp=-1
  Switch{1..8} (8 alike) : Switch  Criteria=u2 ~= 0
  DataOUT : Outport  OutDataTypeStr=uint8
  Signal : Outport  Port=2  OutDataTypeStr=uint8
  ADR_OUT : Outport  Port=3  OutDataTypeStr=uint8
  wires:
  Addr/1 -> Compare To Constant4/1
  Data/1 -> Switch1/1
  Bit Concat1/1 -> Data Type Conversion6/1
  Bit Slice/1 -> Data Type Conversion2/1
  Bit Slice1/1 -> Data Type Conversion3/1
  Bit Slice2/1 -> Data Type Conversion4/1
  Bit Slice3/1 -> Data Type Conversion5/1
  Compare To Constant/1 -> Switch3/3, Logical Operator19/1
  Compare To Constant1/1 -> Switch4/3, Logical Operator20/2
  Compare To Constant2/1 -> Switch5/3, Logical Operator21/1
  Compare To Constant3/1 -> Switch6/3, Logical Operator22/2
  Compare To Constant4/1 -> Switch1/2
  Compare To Constant5/1 -> HDL Counter2/1
  Constant1/1 -> Delay2/1
  Constant2/1 -> Switch2/1
  Constant3/1 -> Switch6/1, Switch5/1, Switch4/1, Switch3/1
  Constant4/1 -> Switch7/1
  Constant5/1 -> Switch7/3
  Constant6/1 -> Switch8/1
  Constant7/1 -> Switch8/3
  Data Type Conversion1/1 -> Logical Operator7/1
  Data Type Conversion2/1 -> Logical Operator2/1, Logical Operator1/1
  Data Type Conversion3/1 -> Logical Operator3/1, Logical Operator1/2
  Data Type Conversion4/1 -> Logical Operator9/1, Logical Operator8/1, Logical Operator6/1, Logical Operator5/2, Logical Operator4/2
  Data Type Conversion5/1 -> Switch6/2, Switch5/2, Switch4/2, Switch3/2, Switch2/2, Logical Operator22/1, Logical Operator21/2, Logical Operator20/1, Logical Operator19/2, Logical Operator18/2, Logical Operator17/2
  Data Type Conversion6/1 -> Signal/1
  Delay/1 -> Logical Operator/2, Delay1/1
  Delay1/1 -> HDL Counter/2
  Delay2/1 -> Logical Operator10/1
  Delay3/1 -> Logical Operator16/1
  HDL Counter/1 -> Compare To Constant5/1
  HDL Counter1/1 -> Compare To Constant3/1, Compare To Constant2/1, Compare To Constant1/1, Compare To Constant/1
  HDL Counter2/1 -> Data Type Conversion1/1
  Logical Operator/1 -> Logical Operator17/1
  Logical Operator1/1 -> Logical Operator18/1
  Logical Operator10/1 -> HDL Counter1/2
  Logical Operator11/1 -> Logical Operator10/2
  Logical Operator12/1 -> Bit Concat1/1
  Logical Operator13/1 -> Logical Operator7/2
  Logical Operator14/1 -> Bit Concat1/3
  Logical Operator15/1 -> Bit Concat1/2
  Logical Operator16/1 -> Logical Operator23/1
  Logical Operator17/1 -> HDL Counter1/1, HDL Counter/1
  Logical Operator18/1 -> SA1/2
  Logical Operator19/1 -> SA3/2, SA2/2
  Logical Operator2/1 -> Switch2/3
  Logical Operator20/1 -> SA4/2
  Logical Operator21/1 -> SA5/2
  Logical Operator22/1 -> SA6/2
  Logical Operator23/1 -> Switch8/2
  Logical Operator3/1 -> Logical Operator2/2
  Logical Operator4/1 -> Logical Operator14/1
  Logical Operator5/1 -> Logical Operator15/1
  Logical Operator6/1 -> Logical Operator13/1
  Logical Operator7/1 -> Bit Concat1/4
  Logical Operator8/1 -> Logical Operator12/1
  Logical Operator9/1 -> Switch7/2, Logical Operator23/2, Logical Operator16/2, Logical Operator11/1, Delay3/1
  SA1/1 -> Logical Operator/1, Delay/1
  SA2/1 -> Logical Operator4/1
  SA3/1 -> Logical Operator5/1
  SA4/1 -> Logical Operator6/2
  SA5/1 -> Logical Operator8/2
  SA6/1 -> Logical Operator9/2
  SA7/1 -> Switch1/3, Bit Slice3/1, Bit Slice2/1, Bit Slice1/1, Bit Slice/1
  Switch1/1 -> SA7/2, SA7/1
  Switch2/1 -> SA1/1
  Switch3/1 -> SA3/1, SA2/1
  Switch4/1 -> SA4/1
  Switch5/1 -> SA5/1
  Switch6/1 -> SA6/1
  Switch7/1 -> DataOUT/1
  Switch8/1 -> ADR_OUT/1

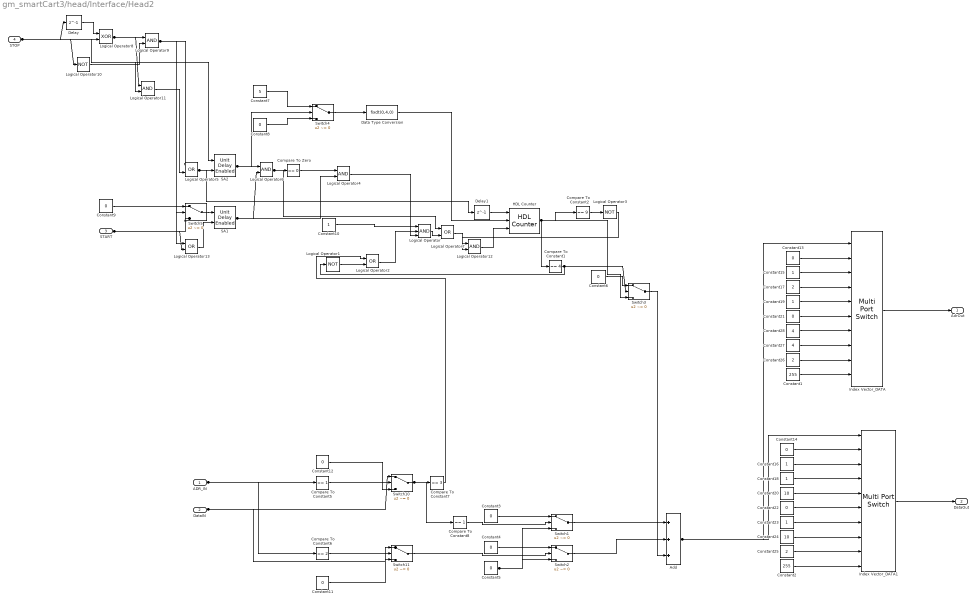
== system gm_smartCart3/head/Interface/Head2 ==
  ADR_IN : Inport  OutDataTypeStr=uint8  SampleTime=1
  DataIN : Inport  Port=2  OutDataTypeStr=uint8  SampleTime=1
  START : Inport  Port=3  OutDataTypeStr=boolean  SampleTime=1
  STOP : Inport  Port=4  OutDataTypeStr=boolean  SampleTime=1
  Add : Sum  Inputs=+++
  Compare To Constant1 : simulink/Logic and Bit Operations/Compare To Constant  relop===  const=4  OutDataTypeStr=boolean
  Compare To Constant2 : simulink/Logic and Bit Operations/Compare To Constant  relop===  const=9  OutDataTypeStr=boolean
  Compare To Constant5 : simulink/Logic and Bit Operations/Compare To Constant  relop===  const=1  OutDataTypeStr=boolean
  Compare To Constant6 : simulink/Logic and Bit Operations/Compare To Constant  relop===  const=2  OutDataTypeStr=boolean
  Compare To Constant7 : simulink/Logic and Bit Operations/Compare To Constant  relop===  const=3  OutDataTypeStr=boolean
  Compare To Constant8 : simulink/Logic and Bit Operations/Compare To Constant  relop===  const=1  OutDataTypeStr=boolean
  Compare To Zero : simulink/Logic and Bit Operations/Compare To Zero  relop===  OutDataTypeStr=boolean
  Constant1 : Constant  Value=255  OutDataTypeStr=uint8
  Constant10 : Constant  OutDataTypeStr=boolean
  Constant{3..6,11..14,21..22} (10 alike) : Constant  Value=0  OutDataTypeStr=uint8
  Constant{15..16,18..19,23} (5 alike) : Constant  OutDataTypeStr=uint8
  Constant17 : Constant  Value=2  OutDataTypeStr=uint8
  Constant2 : Constant  Value=255  OutDataTypeStr=uint8
  Constant20 : Constant  Value=10  OutDataTypeStr=uint8
  Constant24 : Constant  Value=10  OutDataTypeStr=uint8
  Constant25 : Constant  Value=2  OutDataTypeStr=uint8
  Constant26 : Constant  Value=2  OutDataTypeStr=uint8
  Constant27 : Constant  Value=4  OutDataTypeStr=uint8
  Constant28 : Constant  Value=4  OutDataTypeStr=uint8
  Constant7 : Constant  Value=5  OutDataTypeStr=fixdt(0,4,0)
  Constant8 : Constant  Value=0  OutDataTypeStr=fixdt(0,4,0)
  Constant9 : Constant  Value=0  OutDataTypeStr=boolean
  Data Type Conversion : DataTypeConversion  OutDataTypeStr=fixdt(0,4,0)
  Delay : Delay  DelayLength=1  InitialCondition=0
  Delay1 : Delay  DelayLength=1  InitialCondition=0
  HDL Counter : hdlsllib/HDL Operations/HDL Counter  CountType=Free running  CountInit=0  CountStep=1  CountMax=100  CountFromType=Initial value  CountFrom=0  CountResetPort=off  CountLoadPort=on  CountEnbPort=on  CountDirPort=off  CountDataType=Unsigned  CountWordLen=4  CountFracLen=0  CountSampTime=1
  Index Vector_DATA : MultiPortSwitch  DataPortOrder=Zero-based contiguous  Inputs=9  DiagnosticForDefault=None  zeroidx=on  OutDataTypeStr=uint8
  Index Vector_DATA1 : MultiPortSwitch  DataPortOrder=Zero-based contiguous  Inputs=9  DiagnosticForDefault=None  zeroidx=on  OutDataTypeStr=uint8
  Logical Operator : Logic  Inputs=3  AllPortsSameDT=off  OutDataTypeStr=boolean
  Logical Operator1 : Logic  Operator=NOT  AllPortsSameDT=off  OutDataTypeStr=boolean
  Logical Operator10 : Logic  Operator=NOT  AllPortsSameDT=off  OutDataTypeStr=boolean
  Logical Operator{4,6,9,11..12} (5 alike) : Logic  AllPortsSameDT=off  OutDataTypeStr=boolean
  Logical Operator{2,5,7,13} (4 alike) : Logic  Operator=OR  AllPortsSameDT=off  OutDataTypeStr=boolean
  Logical Operator3 : Logic  Operator=NOT  AllPortsSameDT=off  OutDataTypeStr=boolean
  Logical Operator8 : Logic  Operator=XOR  AllPortsSameDT=off  OutDataTypeStr=boolean
  SA1 : simulink/Additional Math & Discrete/Additional Discrete/Unit Delay Enabled  vinit=0  tsamp=-1
  SA2 : simulink/Additional Math & Discrete/Additional Discrete/Unit Delay Enabled  vinit=0  tsamp=-1
  Switch{1..5,10..11} (7 alike) : Switch  Criteria=u2 ~= 0  OutDataTypeStr=uint8
  AdrOut : Outport  OutDataTypeStr=uint8
  DataOut : Outport  Port=2  OutDataTypeStr=uint8
  wires:
  ADR_IN/1 -> Compare To Constant6/1, Compare To Constant5/1
  DataIN/1 -> Switch11/1, Switch10/1
  START/1 -> Switch5/3, Logical Operator13/2
  STOP/1 -> Logical Operator8/2, Logical Operator11/2, Logical Operator10/1, SA2/1, Delay/1
  Add/1 -> Index Vector_DATA1/1, Index Vector_DATA/1
  Compare To Constant1/1 -> Switch3/2, Logical Operator1/1
  Compare To Constant2/1 -> Logical Operator3/1
  Compare To Constant5/1 -> Switch10/2
  Compare To Constant6/1 -> Switch11/2
  Compare To Constant7/1 -> Logical Operator2/1
  Compare To Constant8/1 -> Switch1/2
  Compare To Zero/1 -> Logical Operator4/1
  Constant1/1 -> Index Vector_DATA/10
  Constant10/1 -> Logical Operator/1
  Constant11/1 -> Switch11/3
  Constant12/1 -> Switch10/3
  Constant13/1 -> Index Vector_DATA/2
  Constant14/1 -> Index Vector_DATA1/2
  Constant15/1 -> Index Vector_DATA/3
  Constant16/1 -> Index Vector_DATA1/3
  Constant17/1 -> Index Vector_DATA/4
  Constant18/1 -> Index Vector_DATA1/4
  Constant19/1 -> Index Vector_DATA/5
  Constant2/1 -> Index Vector_DATA1/10
  Constant20/1 -> Index Vector_DATA1/5
  Constant21/1 -> Index Vector_DATA/6
  Constant22/1 -> Index Vector_DATA1/6
  Constant23/1 -> Index Vector_DATA1/7
  Constant24/1 -> Index Vector_DATA1/8
  Constant25/1 -> Index Vector_DATA1/9
  Constant26/1 -> Index Vector_DATA/9
  Constant27/1 -> Index Vector_DATA/8
  Constant28/1 -> Index Vector_DATA/7
  Constant3/1 -> Switch1/1
  Constant4/1 -> Switch2/1
  Constant5/1 -> Switch2/3, Switch1/3
  Constant6/1 -> Switch3/1
  Constant7/1 -> Switch4/1
  Constant8/1 -> Switch4/3
  Constant9/1 -> Switch5/1
  Data Type Conversion/1 -> HDL Counter/2
  Delay/1 -> Logical Operator8/1
  Delay1/1 -> HDL Counter/1
  HDL Counter/1 -> Switch3/3, Compare To Constant2/1, Compare To Constant1/1
  Index Vector_DATA/1 -> AdrOut/1
  Index Vector_DATA1/1 -> DataOut/1
  Logical Operator/1 -> Logical Operator7/2
  Logical Operator1/1 -> Logical Operator2/2
  Logical Operator10/1 -> Logical Operator9/2
  Logical Operator11/1 -> Logical Operator5/2
  Logical Operator12/1 -> HDL Counter/3
  Logical Operator13/1 -> SA1/2
  Logical Operator2/1 -> Logical Operator/2
  Logical Operator3/1 -> Logical Operator12/2
  Logical Operator4/1 -> Logical Operator/3
  Logical Operator5/1 -> SA2/2, Delay1/1
  Logical Operator6/1 -> Logical Operator7/1, Compare To Zero/1
  Logical Operator7/1 -> Logical Operator12/1
  Logical Operator8/1 -> Logical Operator9/1, Logical Operator11/1
  Logical Operator9/1 -> Switch5/2, Logical Operator5/1, Logical Operator13/1
  SA1/1 -> Logical Operator6/2, Logical Operator4/2
  SA2/1 -> Switch4/2, Logical Operator6/1
  Switch1/1 -> Add/1
  Switch10/1 -> Compare To Constant8/1, Compare To Constant7/1
  Switch11/1 -> Switch2/2
  Switch2/1 -> Add/2
  Switch3/1 -> Add/3
  Switch4/1 -> Data Type Conversion/1
  Switch5/1 -> SA1/1

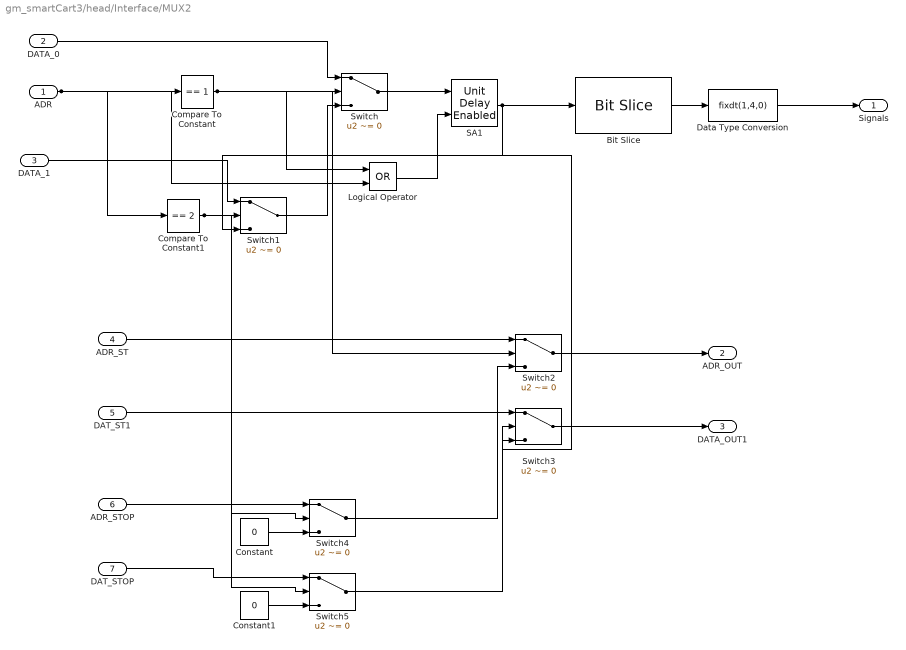
== system gm_smartCart3/head/Interface/MUX2 ==
  ADR : Inport  OutDataTypeStr=uint8  SampleTime=1
  DATA_0 : Inport  Port=2  OutDataTypeStr=uint8  SampleTime=1
  DATA_1 : Inport  Port=3  OutDataTypeStr=uint8  SampleTime=1
  ADR_ST : Inport  Port=4  OutDataTypeStr=uint8  SampleTime=1
  DAT_ST1 : Inport  Port=5  OutDataTypeStr=uint8  SampleTime=1
  ADR_STOP : Inport  Port=6  OutDataTypeStr=uint8  SampleTime=1
  DAT_STOP : Inport  Port=7  OutDataTypeStr=uint8  SampleTime=1
  Bit Slice : hdlsllib/HDL Operations/Bit Slice  lidx=4  ridx=0
  Compare To Constant : simulink/Logic and Bit Operations/Compare To Constant  relop===  const=1  OutDataTypeStr=boolean
  Compare To Constant1 : simulink/Logic and Bit Operations/Compare To Constant  relop===  const=2  OutDataTypeStr=boolean
  Constant : Constant  Value=0  OutDataTypeStr=boolean
  Constant1 : Constant  Value=0  OutDataTypeStr=boolean
  Data Type Conversion : DataTypeConversion  OutDataTypeStr=fixdt(1,4,0)
  Logical Operator : Logic  Operator=OR  AllPortsSameDT=off  OutDataTypeStr=boolean
  SA1 : simulink/Additional Math & Discrete/Additional Discrete/Unit Delay Enabled  vinit=0  tsamp=-1
  Switch{,1..5} (6 alike) : Switch  Criteria=u2 ~= 0  OutDataTypeStr=uint8
  Signals : Outport  OutDataTypeStr=fixdt(1,4,0)
  ADR_OUT : Outport  Port=2  OutDataTypeStr=uint8
  DATA_OUT1 : Outport  Port=3  OutDataTypeStr=uint8
  wires:
  ADR/1 -> Logical Operator/2, Compare To Constant1/1, Compare To Constant/1
  DATA_0/1 -> Switch/1
  DATA_1/1 -> Switch1/1
  ADR_ST/1 -> Switch2/1
  DAT_ST1/1 -> Switch3/1
  ADR_STOP/1 -> Switch4/1
  DAT_STOP/1 -> Switch5/1
  Bit Slice/1 -> Data Type Conversion/1
  Compare To Constant/1 -> Switch3/2, Switch2/2, Switch/2, Logical Operator/1
  Compare To Constant1/1 -> Switch5/2, Switch4/2, Switch1/2
  Constant/1 -> Switch4/3
  Constant1/1 -> Switch5/3
  Data Type Conversion/1 -> Signals/1
  Logical Operator/1 -> SA1/2
  SA1/1 -> Switch1/3, Bit Slice/1
  Switch/1 -> SA1/1
  Switch1/1 -> Switch/3
  Switch2/1 -> ADR_OUT/1
  Switch3/1 -> DATA_OUT1/1
  Switch4/1 -> Switch2/3
  Switch5/1 -> Switch3/3

== system gm_smartCart3/head/Interface/Swith_signal2 ==
  Adr : Inport  OutDataTypeStr=uint8  SampleTime=1
  Data : Inport  Port=2  OutDataTypeStr=uint8  SampleTime=1
  Compare To Constant : simulink/Logic and Bit Operations/Compare To Constant  relop===  const=2  OutDataTypeStr=boolean
  SA1 : simulink/Additional Math & Discrete/Additional Discrete/Unit Delay Enabled  vinit=0  tsamp=-1
  OutAddr : Outport  OutDataTypeStr=uint8
  wires:
  Adr/1 -> Compare To Constant/1
  Data/1 -> SA1/1
  Compare To Constant/1 -> SA1/2
  SA1/1 -> OutAddr/1

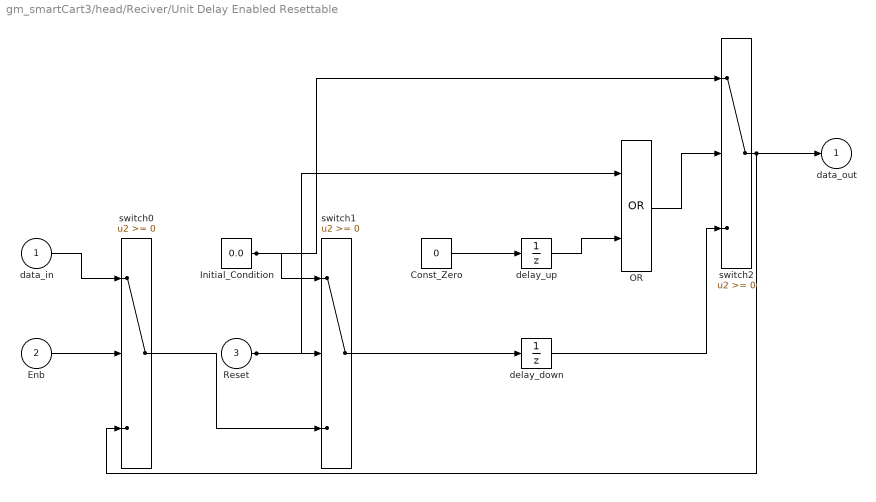
== system gm_smartCart3/head/Reciver/Unit Delay Enabled Resettable ==
  data_in : Inport
  Enb : Inport  Port=2
  Reset : Inport  Port=3
  Const_Zero : Constant  Value=0  OutDataTypeStr=boolean
  Initial_Condition : Constant  Value=0.0  OutDataTypeStr=Inherit: Inherit via back propagation
  OR : Logic  Operator=OR
  delay_down : UnitDelay  SampleTime=-1
  delay_up : UnitDelay  InitialCondition=1  SampleTime=-1
  switch0 : Switch  SaturateOnIntegerOverflow=on  InputSameDT=on
  switch1 : Switch  SaturateOnIntegerOverflow=on  InputSameDT=on
  switch2 : Switch  SaturateOnIntegerOverflow=on  InputSameDT=on
  data_out : Outport
  wires:
  data_in/1 -> switch0/1
  Enb/1 -> switch0/2
  switch2/1 -> switch0/3, data_out/1
  Initial_Condition/1 -> switch1/1, switch2/1
  Reset/1 -> switch1/2, OR/1
  switch0/1 -> switch1/3
  Const_Zero/1 -> delay_up/1
  switch1/1 -> delay_down/1
  delay_up/1 -> OR/2
  OR/1 -> switch2/2
  delay_down/1 -> switch2/3

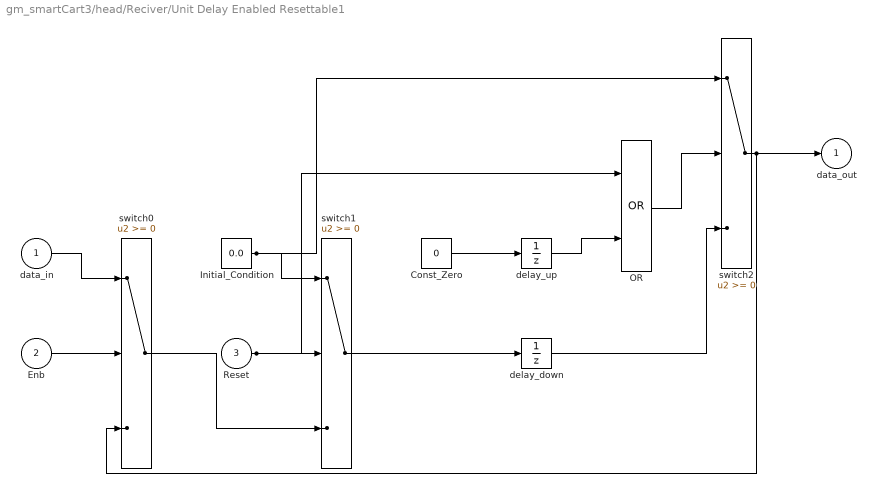
== system gm_smartCart3/head/Reciver/Unit Delay Enabled Resettable1 ==
  data_in : Inport
  Enb : Inport  Port=2
  Reset : Inport  Port=3
  Const_Zero : Constant  Value=0  OutDataTypeStr=boolean
  Initial_Condition : Constant  Value=0.0  OutDataTypeStr=Inherit: Inherit via back propagation
  OR : Logic  Operator=OR
  delay_down : UnitDelay  SampleTime=-1
  delay_up : UnitDelay  InitialCondition=1  SampleTime=-1
  switch0 : Switch  SaturateOnIntegerOverflow=on  InputSameDT=on
  switch1 : Switch  SaturateOnIntegerOverflow=on  InputSameDT=on
  switch2 : Switch  SaturateOnIntegerOverflow=on  InputSameDT=on
  data_out : Outport
  wires:
  data_in/1 -> switch0/1
  Enb/1 -> switch0/2
  switch2/1 -> switch0/3, data_out/1
  Initial_Condition/1 -> switch1/1, switch2/1
  Reset/1 -> switch1/2, OR/1
  switch0/1 -> switch1/3
  Const_Zero/1 -> delay_up/1
  switch1/1 -> delay_down/1
  delay_up/1 -> OR/2
  OR/1 -> switch2/2
  delay_down/1 -> switch2/3

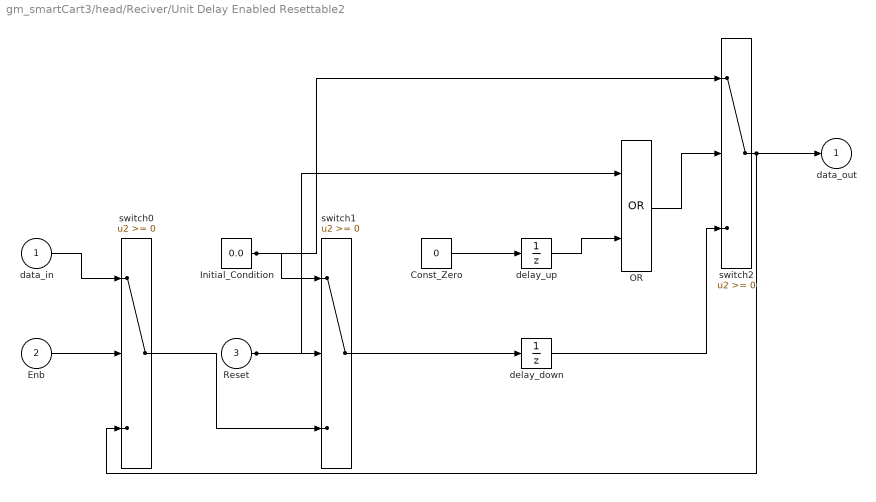
== system gm_smartCart3/head/Reciver/Unit Delay Enabled Resettable2 ==
  data_in : Inport
  Enb : Inport  Port=2
  Reset : Inport  Port=3
  Const_Zero : Constant  Value=0  OutDataTypeStr=boolean
  Initial_Condition : Constant  Value=0.0  OutDataTypeStr=Inherit: Inherit via back propagation
  OR : Logic  Operator=OR
  delay_down : UnitDelay  SampleTime=-1
  delay_up : UnitDelay  InitialCondition=1  SampleTime=-1
  switch0 : Switch  SaturateOnIntegerOverflow=on  InputSameDT=on
  switch1 : Switch  SaturateOnIntegerOverflow=on  InputSameDT=on
  switch2 : Switch  SaturateOnIntegerOverflow=on  InputSameDT=on
  data_out : Outport
  wires:
  data_in/1 -> switch0/1
  Enb/1 -> switch0/2
  switch2/1 -> switch0/3, data_out/1
  Initial_Condition/1 -> switch1/1, switch2/1
  Reset/1 -> switch1/2, OR/1
  switch0/1 -> switch1/3
  Const_Zero/1 -> delay_up/1
  switch1/1 -> delay_down/1
  delay_up/1 -> OR/2
  OR/1 -> switch2/2
  delay_down/1 -> switch2/3

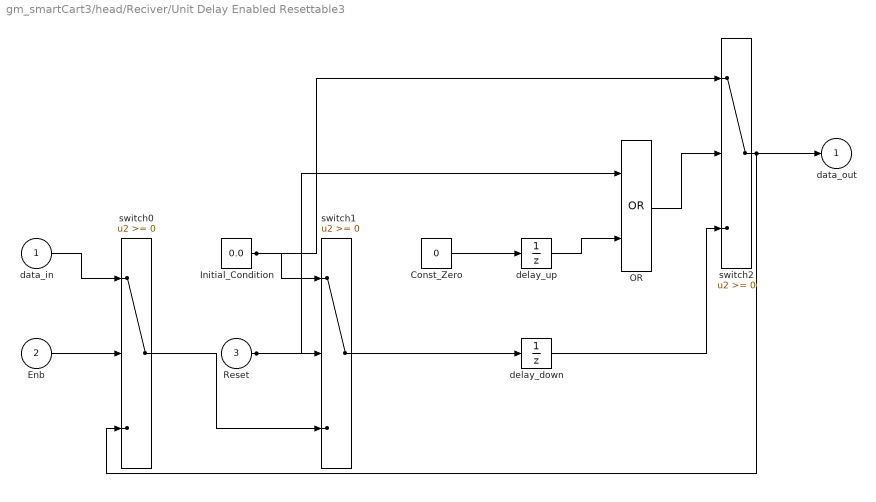
== system gm_smartCart3/head/Reciver/Unit Delay Enabled Resettable3 ==
  data_in : Inport
  Enb : Inport  Port=2
  Reset : Inport  Port=3
  Const_Zero : Constant  Value=0  OutDataTypeStr=boolean
  Initial_Condition : Constant  Value=0.0  OutDataTypeStr=Inherit: Inherit via back propagation
  OR : Logic  Operator=OR
  delay_down : UnitDelay  SampleTime=-1
  delay_up : UnitDelay  InitialCondition=1  SampleTime=-1
  switch0 : Switch  SaturateOnIntegerOverflow=on  InputSameDT=on
  switch1 : Switch  SaturateOnIntegerOverflow=on  InputSameDT=on
  switch2 : Switch  SaturateOnIntegerOverflow=on  InputSameDT=on
  data_out : Outport
  wires:
  data_in/1 -> switch0/1
  Enb/1 -> switch0/2
  switch2/1 -> switch0/3, data_out/1
  Initial_Condition/1 -> switch1/1, switch2/1
  Reset/1 -> switch1/2, OR/1
  switch0/1 -> switch1/3
  Const_Zero/1 -> delay_up/1
  switch1/1 -> delay_down/1
  delay_up/1 -> OR/2
  OR/1 -> switch2/2
  delay_down/1 -> switch2/3

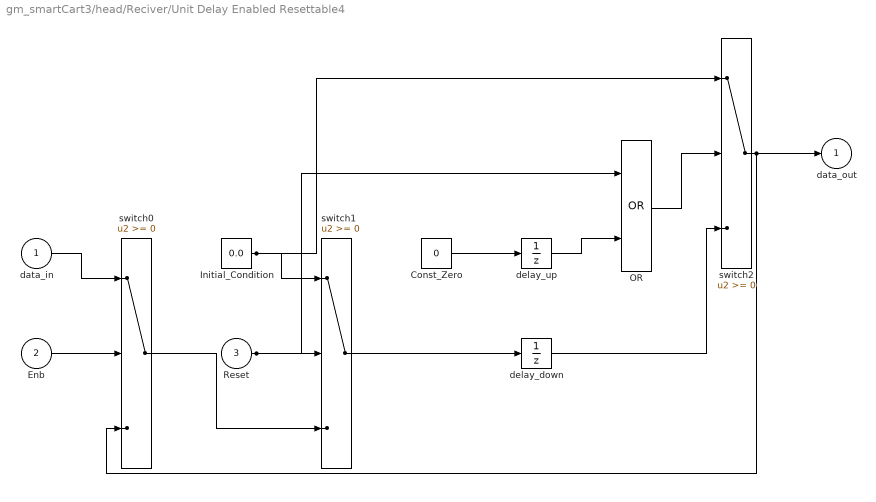
== system gm_smartCart3/head/Reciver/Unit Delay Enabled Resettable4 ==
  data_in : Inport
  Enb : Inport  Port=2
  Reset : Inport  Port=3
  Const_Zero : Constant  Value=0  OutDataTypeStr=boolean
  Initial_Condition : Constant  Value=0.0  OutDataTypeStr=Inherit: Inherit via back propagation
  OR : Logic  Operator=OR
  delay_down : UnitDelay  SampleTime=-1
  delay_up : UnitDelay  InitialCondition=1  SampleTime=-1
  switch0 : Switch  SaturateOnIntegerOverflow=on  InputSameDT=on
  switch1 : Switch  SaturateOnIntegerOverflow=on  InputSameDT=on
  switch2 : Switch  SaturateOnIntegerOverflow=on  InputSameDT=on
  data_out : Outport
  wires:
  data_in/1 -> switch0/1
  Enb/1 -> switch0/2
  switch2/1 -> switch0/3, data_out/1
  Initial_Condition/1 -> switch1/1, switch2/1
  Reset/1 -> switch1/2, OR/1
  switch0/1 -> switch1/3
  Const_Zero/1 -> delay_up/1
  switch1/1 -> delay_down/1
  delay_up/1 -> OR/2
  OR/1 -> switch2/2
  delay_down/1 -> switch2/3

== system gm_smartCart3/head/Reciver/Unit Delay Enabled Resettable5 ==
  data_in : Inport
  Enb : Inport  Port=2
  Reset : Inport  Port=3
  Const_Zero : Constant  Value=0  OutDataTypeStr=boolean
  Initial_Condition : Constant  Value=0.0  OutDataTypeStr=Inherit: Inherit via back propagation
  OR : Logic  Operator=OR
  delay_down : UnitDelay  SampleTime=-1
  delay_up : UnitDelay  InitialCondition=1  SampleTime=-1
  switch0 : Switch  SaturateOnIntegerOverflow=on  InputSameDT=on
  switch1 : Switch  SaturateOnIntegerOverflow=on  InputSameDT=on
  switch2 : Switch  SaturateOnIntegerOverflow=on  InputSameDT=on
  data_out : Outport
  wires:
  data_in/1 -> switch0/1
  Enb/1 -> switch0/2
  switch2/1 -> switch0/3, data_out/1
  Initial_Condition/1 -> switch1/1, switch2/1
  Reset/1 -> switch1/2, OR/1
  switch0/1 -> switch1/3
  Const_Zero/1 -> delay_up/1
  switch1/1 -> delay_down/1
  delay_up/1 -> OR/2
  OR/1 -> switch2/2
  delay_down/1 -> switch2/3

== system gm_smartCart3/head/Reciver/Unit Delay Enabled Resettable6 ==
  data_in : Inport
  Enb : Inport  Port=2
  Reset : Inport  Port=3
  Const_Zero : Constant  Value=0  OutDataTypeStr=boolean
  Initial_Condition : Constant  Value=0.0  OutDataTypeStr=Inherit: Inherit via back propagation
  OR : Logic  Operator=OR
  delay_down : UnitDelay  SampleTime=-1
  delay_up : UnitDelay  InitialCondition=1  SampleTime=-1
  switch0 : Switch  SaturateOnIntegerOverflow=on  InputSameDT=on
  switch1 : Switch  SaturateOnIntegerOverflow=on  InputSameDT=on
  switch2 : Switch  SaturateOnIntegerOverflow=on  InputSameDT=on
  data_out : Outport
  wires:
  data_in/1 -> switch0/1
  Enb/1 -> switch0/2
  switch2/1 -> switch0/3, data_out/1
  Initial_Condition/1 -> switch1/1, switch2/1
  Reset/1 -> switch1/2, OR/1
  switch0/1 -> switch1/3
  Const_Zero/1 -> delay_up/1
  switch1/1 -> delay_down/1
  delay_up/1 -> OR/2
  OR/1 -> switch2/2
  delay_down/1 -> switch2/3

== system gm_smartCart3/head/Reciver/Unit Delay Enabled Resettable7 ==
  data_in : Inport
  Enb : Inport  Port=2
  Reset : Inport  Port=3
  Const_Zero : Constant  Value=0  OutDataTypeStr=boolean
  Initial_Condition : Constant  Value=0.0  OutDataTypeStr=Inherit: Inherit via back propagation
  OR : Logic  Operator=OR
  delay_down : UnitDelay  SampleTime=-1
  delay_up : UnitDelay  InitialCondition=1  SampleTime=-1
  switch0 : Switch  SaturateOnIntegerOverflow=on  InputSameDT=on
  switch1 : Switch  SaturateOnIntegerOverflow=on  InputSameDT=on
  switch2 : Switch  SaturateOnIntegerOverflow=on  InputSameDT=on
  data_out : Outport
  wires:
  data_in/1 -> switch0/1
  Enb/1 -> switch0/2
  switch2/1 -> switch0/3, data_out/1
  Initial_Condition/1 -> switch1/1, switch2/1
  Reset/1 -> switch1/2, OR/1
  switch0/1 -> switch1/3
  Const_Zero/1 -> delay_up/1
  switch1/1 -> delay_down/1
  delay_up/1 -> OR/2
  OR/1 -> switch2/2
  delay_down/1 -> switch2/3

== system gm_smartCart3/head/Reciver/Unit Delay Enabled Resettable8 ==
  data_in : Inport
  Enb : Inport  Port=2
  Reset : Inport  Port=3
  Const_Zero : Constant  Value=0  OutDataTypeStr=boolean
  Initial_Condition : Constant  Value=0.0  OutDataTypeStr=Inherit: Inherit via back propagation
  OR : Logic  Operator=OR
  delay_down : UnitDelay  SampleTime=-1
  delay_up : UnitDelay  InitialCondition=1  SampleTime=-1
  switch0 : Switch  SaturateOnIntegerOverflow=on  InputSameDT=on
  switch1 : Switch  SaturateOnIntegerOverflow=on  InputSameDT=on
  switch2 : Switch  SaturateOnIntegerOverflow=on  InputSameDT=on
  data_out : Outport
  wires:
  data_in/1 -> switch0/1
  Enb/1 -> switch0/2
  switch2/1 -> switch0/3, data_out/1
  Initial_Condition/1 -> switch1/1, switch2/1
  Reset/1 -> switch1/2, OR/1
  switch0/1 -> switch1/3
  Const_Zero/1 -> delay_up/1
  switch1/1 -> delay_down/1
  delay_up/1 -> OR/2
  OR/1 -> switch2/2
  delay_down/1 -> switch2/3
